simulink model "Cluster_HMI"  (R2024a)
settings: Solver=VariableStepAuto  StartTime=0.0  StopTime=10.0  RelTol=1e-3
libraries: simulink x1, spsMonostableLib x1
settings Model: Creator=henri  LastModifiedBy=henri

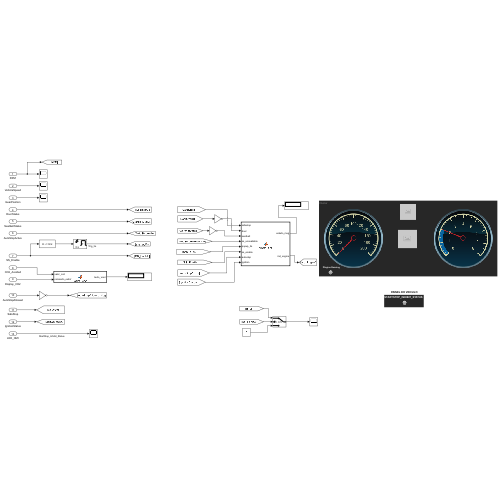
[thumbnail: Simulink's stored preview of the top-level diagram]
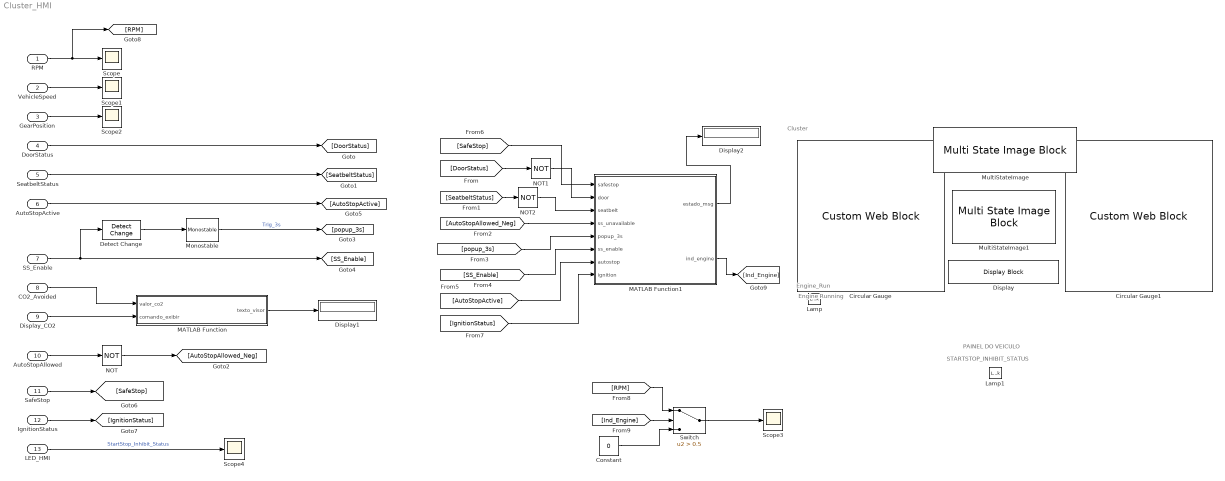
== system Cluster_HMI ==
  note: Engine Running
  note: STARTSTOP_INHIBIT_STATUS
  note: Engine_Run
  note: Cluster
  note: PAINEL DO VEICULO
  RPM : Inport  RequirementInfo={} %GIDa_701cb9d7_1c6a_4930_8ae1_c3f9a837b0c9
  VehicleSpeed : Inport  RequirementInfo={} %GIDa_2d9c3a77_c6f6_418b_8e13_68813d5ea9b5  Port=2
  GearPosition : Inport  RequirementInfo={} %GIDa_c6ce69f4_9c31_429f_b9bc_75ef1a17d6ed  Port=3
  DoorStatus : Inport  RequirementInfo={} %GIDa_d72df632_89b1_4396_adeb_ebc89bf69c51  Port=4
  SeatbeltStatus : Inport  RequirementInfo={} %GIDa_18d845fd_3170_430e_97dc_0ac91aff9f15  Port=5
  AutoStopActive : Inport  RequirementInfo={} %GIDa_37518f2b_e752_4b1f_8c46_cfe48663f65d  Port=6
  SS_Enable : Inport  RequirementInfo={} %GIDa_10efa209_da12_4e26_ab38_1e39670f885c  Port=7
  CO2_Avoided : Inport  RequirementInfo={} %GIDa_176e85e5_0be0_4fa3_869e_c19e09e86116  Port=8
  Display_CO2 : Inport  RequirementInfo={} %GIDa_b6f97d48_dcb8_4ba0_b3dc_e52b49ed6545  Port=9
  AutoStopAllowed : Inport  RequirementInfo={} %GIDa_274fdb3f_b9e4_413b_891d_ddf4024beb1a  Port=10
  SafeStop : Inport  RequirementInfo={} %GIDa_2abc3005_5b3a_47dc_bfb2_0f18a82977d9  Port=11
  IgnitionStatus : Inport  RequirementInfo={} %GIDa_800ccd42_76b0_45b4_b5ac_9e6254392555  Port=12
  LED_HMI : Inport  RequirementInfo={} %GIDa_c1088d5e_6a51_4c66_ba2d_65ca3d813fbb  Port=13
  Circular Gauge : CustomWebBlock  RequirementInfo={} %GIDa_7b8fb6d0_a955_42f4_bee6_c529bf727d9c  LabelPosition=Hide  ShowInitialText=on  Configuration="{\"components\":[{\"name\":\"CircularScaleComponent\",\"settings\":{\"bounds\":{\"max\":200,\"min\":0,\"tickInterval\":20},\"direction\":\"cw\",\"flipLimits\":0,\"innerRadius\":0.75,\"internalTickHeightScaleFactor\":1,\"labelColor\":[255,255,200],\"labelFont\":{\"font\":\"Arial\",\"fontSize\":12},\"labelRadius\":0.528,\"labelTransparency\":1,\"minorTickHeightScaleFactor\":0.2,\"needleImage\":{\"size\":[200,50],\"src\":\"data:image\\/svg+xml;base64,PD94bWwgdmVyc2lvbj0iMS4wIiBlbmNvZGluZz0idXRmLTgiPz4KPCEtLSBHZW5lcmF0b3I6IEFkb2JlIElsbHVzdHJhdG9yIDI0LjEuMiwgU1ZHIEV4cG9ydCBQbHVnLUluIC4gU1ZHIFZlcnNpb246IDYuMDAgQnVpbGQgMCkgIC0tPgo8c3ZnIHZlcnNpb249IjEuMSIgaWQ9IkxheWVyXzEiIHhtbG5zPSJodHRwOi8vd3d3LnczLm9yZy8yMDAwL3N2ZyIgeG1sbnM6eGxpbms9Imh0dHA6Ly93d3cudzMub3JnLzE5OTkveGxpbmsiIHg9IjBweCIgeT0iMHB4IgoJIHZpZXdCb3g9IjAgMCAyMDAgNTAiIHN0eWxlPSJlbmFibGUtYmFja2dyb3VuZDpuZXcgMCAwIDIwMCA1MDsiIHhtbDpzcGFjZT0icHJlc2VydmUiPgo8c3R5bGUgdHlwZT0idGV4dC9jc3MiPgoJLnN0MHtmaWxsOiNFQzIxMjc7fQo8L3N0eWxlPgo8cGF0aCBjbGFzcz0ic3QwIiBkPSJNMTYyLjgsMTMuN0MxNjksNC40LDE4MS43LDEuOSwxOTEsOC4xczExLjgsMTguOSw1LjYsMjguMnMtMTguOSwxMS44LTI4LjIsNS42bDAsMAoJQzE1OS4xLDM1LjYsMTU2LjYsMjMsMTYyLjgsMTMuN0wxNjIuOCwxMy43eiBNMTY1LjgsMTUuOGMtNS4xLDcuNi0zLjEsMTcuOSw0LjYsMjNjNy42LDUuMSwxNy45LDMuMSwyMy00LjYKCWM1LjEtNy42LDMuMS0xNy45LTQuNi0yM2wwLDBDMTgxLjIsNi4yLDE3MC45LDguMiwxNjUuOCwxNS44eiIvPgo8cGF0aCBjbGFzcz0ic3QwIiBkPSJNMC40LDI1Ljl2LTMuM2wxNTktMi41Yy0wLjcsMi42LTAuNyw1LjIsMCw3LjhMMC40LDI1Ljl6Ii8+CjxjaXJjbGUgY2xhc3M9InN0MCIgY3g9IjE3OS42IiBjeT0iMjQiIHI9IjAuNyIvPgo8L3N2Zz4K\"},\"needleOffset\":[0.18464878250906522,0],\"needleOrientation\":-45,\"needleRotation\":180,\"needleSize\":{\"height\":0.11741692305346914,\"width\":0.46108337545091255},\"outerRadius\":0.9,\"position\":[0.05,0.05,0.9,0.9],\"referencePoint\":\"auto\",\"scaleAngle\":270,\"scaleAngleOffset\":135,\"scaleColors\":[],\"scaleColorsSize\":0.2,\"scaleDirection\":\"CW\",\"scalePosition\":[0,0,1,1],\"showLabels\":1,\"showMinorTicks\":1,\"showSpanLine\":1,\"showTicks\":1,\"tickColor\":[252,252,197],\"tickTransparency\":1,\"valueBarColor\":[0,114,189],\"valueBarPosition\":[0,0,1,1],\"valueBarSize\":0.2,\"valueBarTransparency\":1}},{\"name\":\"BackgroundImageComponent\",\"settings\":{\"image\":{\"size\":[500,500],\"src\":\"data:image\\/svg+xml;base64,PD94bWwgdmVyc2lvbj0iMS4wIiBlbmNvZGluZz0iVVRGLTgiIHN0YW5kYWxvbmU9Im5vIj8+CjxzdmcKICAgeG1sbnM6ZGM9Imh0dHA6Ly9wdXJsLm9yZy9kYy9lbGVtZW50cy8xLjEvIgogICB4bWxuczpjYz0iaHR0cDovL2NyZWF0aXZlY29tbW9ucy5vcmcvbnMjIgogICB4bWxuczpyZGY9Imh0dHA6Ly93d3cudzMub3JnLzE5OTkvMDIvMjItcmRmLXN5bnRheC1ucyMiCiAgIHhtbG5zOnN2Zz0iaHR0cDovL3d3dy53My5vcmcvMjAwMC9zdmciCiAgIHhtbG5zPSJodHRwOi8vd3d3LnczLm9yZy8yMDAwL3N2ZyIKICAgeG1sbnM6 ...(+9964 chars)\"},\"position\":[0,0,1,1],\"scaleMode\":\"0\"}},{\"name\":\"ForegroundImageComponent\",\"settings\":{\"image\":{\"size\":[0,0],\"src\":\"default\",\"srcOrientation\":[]},\"isForeground\":1,\"position\":[0,0,1,1],\"scaleMode\":\"0\"}}],\"settings\":{\"BindingType\":\"signal\",\"aspectRatio\":1.032258064516129,\"backgroundColor\":[0,0,0,\"1\"],\"backgroundOffset\":1,\"backgroundOpacity\":1,\"direction\":\"cw\",\"fixedAspectRatio\":\"on\",\"flipLimits\":0,\"orientation\":\"horizontal\",\"showBackgroundColor\":false,\"value\":0,\"version\":\"R2023a\"},\"type\":\"CircularGauge\"}"
  Circular Gauge1 : CustomWebBlock  RequirementInfo={} %GIDa_e85ea3ac_6d53_4628_b3b0_ac8b9261904e  LabelPosition=Hide  ShowInitialText=on  Configuration="{\"components\":[{\"name\":\"CircularScaleComponent\",\"settings\":{\"bounds\":{\"max\":8,\"min\":0,\"tickInterval\":1},\"direction\":\"cw\",\"flipLimits\":0,\"innerRadius\":0.75,\"internalTickHeightScaleFactor\":1,\"labelColor\":[255,255,200],\"labelFont\":{\"font\":\"Arial\",\"fontSize\":12},\"labelRadius\":0.528,\"labelTransparency\":1,\"minorTickHeightScaleFactor\":0.2,\"needleImage\":{\"size\":[200,50],\"src\":\"data:image\\/svg+xml;base64,PD94bWwgdmVyc2lvbj0iMS4wIiBlbmNvZGluZz0idXRmLTgiPz4KPCEtLSBHZW5lcmF0b3I6IEFkb2JlIElsbHVzdHJhdG9yIDI0LjEuMiwgU1ZHIEV4cG9ydCBQbHVnLUluIC4gU1ZHIFZlcnNpb246IDYuMDAgQnVpbGQgMCkgIC0tPgo8c3ZnIHZlcnNpb249IjEuMSIgaWQ9IkxheWVyXzEiIHhtbG5zPSJodHRwOi8vd3d3LnczLm9yZy8yMDAwL3N2ZyIgeG1sbnM6eGxpbms9Imh0dHA6Ly93d3cudzMub3JnLzE5OTkveGxpbmsiIHg9IjBweCIgeT0iMHB4IgoJIHZpZXdCb3g9IjAgMCAyMDAgNTAiIHN0eWxlPSJlbmFibGUtYmFja2dyb3VuZDpuZXcgMCAwIDIwMCA1MDsiIHhtbDpzcGFjZT0icHJlc2VydmUiPgo8c3R5bGUgdHlwZT0idGV4dC9jc3MiPgoJLnN0MHtmaWxsOiNFQzIxMjc7fQo8L3N0eWxlPgo8cGF0aCBjbGFzcz0ic3QwIiBkPSJNMTYyLjgsMTMuN0MxNjksNC40LDE4MS43LDEuOSwxOTEsOC4xczExLjgsMTguOSw1LjYsMjguMnMtMTguOSwxMS44LTI4LjIsNS42bDAsMAoJQzE1OS4xLDM1LjYsMTU2LjYsMjMsMTYyLjgsMTMuN0wxNjIuOCwxMy43eiBNMTY1LjgsMTUuOGMtNS4xLDcuNi0zLjEsMTcuOSw0LjYsMjNjNy42LDUuMSwxNy45LDMuMSwyMy00LjYKCWM1LjEtNy42LDMuMS0xNy45LTQuNi0yM2wwLDBDMTgxLjIsNi4yLDE3MC45LDguMiwxNjUuOCwxNS44eiIvPgo8cGF0aCBjbGFzcz0ic3QwIiBkPSJNMC40LDI1Ljl2LTMuM2wxNTktMi41Yy0wLjcsMi42LTAuNyw1LjIsMCw3LjhMMC40LDI1Ljl6Ii8+CjxjaXJjbGUgY2xhc3M9InN0MCIgY3g9IjE3OS42IiBjeT0iMjQiIHI9IjAuNyIvPgo8L3N2Zz4K\"},\"needleOffset\":[0.18464878250906522,0],\"needleOrientation\":-45,\"needleRotation\":180,\"needleSize\":{\"height\":0.11741692305346914,\"width\":0.46108337545091255},\"outerRadius\":0.9,\"position\":[0.05,0.05,0.9,0.9],\"referencePoint\":\"auto\",\"scaleAngle\":270,\"scaleAngleOffset\":135,\"scaleColors\":[],\"scaleColorsSize\":0.2,\"scaleDirection\":\"CW\",\"scalePosition\":[0,0,1,1],\"showLabels\":1,\"showMinorTicks\":1,\"showSpanLine\":1,\"showTicks\":1,\"tickColor\":[252,252,197],\"tickTransparency\":1,\"valueBarColor\":[0,114,189],\"valueBarPosition\":[0,0,1,1],\"valueBarSize\":0.2,\"valueBarTransparency\":1}},{\"name\":\"BackgroundImageComponent\",\"settings\":{\"image\":{\"size\":[500,500],\"src\":\"data:image\\/svg+xml;base64,PD94bWwgdmVyc2lvbj0iMS4wIiBlbmNvZGluZz0iVVRGLTgiIHN0YW5kYWxvbmU9Im5vIj8+CjxzdmcKICAgeG1sbnM6ZGM9Imh0dHA6Ly9wdXJsLm9yZy9kYy9lbGVtZW50cy8xLjEvIgogICB4bWxuczpjYz0iaHR0cDovL2NyZWF0aXZlY29tbW9ucy5vcmcvbnMjIgogICB4bWxuczpyZGY9Imh0dHA6Ly93d3cudzMub3JnLzE5OTkvMDIvMjItcmRmLXN5bnRheC1ucyMiCiAgIHhtbG5zOnN2Zz0iaHR0cDovL3d3dy53My5vcmcvMjAwMC9zdmciCiAgIHhtbG5zPSJodHRwOi8vd3d3LnczLm9yZy8yMDAwL3N2ZyIKICAgeG1sbnM6 ...(+9964 chars)\"},\"position\":[0,0,1,1],\"scaleMode\":\"0\"}},{\"name\":\"ForegroundImageComponent\",\"settings\":{\"image\":{\"size\":[0,0],\"src\":\"default\",\"srcOrientation\":[]},\"isForeground\":1,\"position\":[0,0,1,1],\"scaleMode\":\"0\"}}],\"settings\":{\"BindingType\":\"signal\",\"aspectRatio\":1.032258064516129,\"backgroundColor\":[0,0,0,\"1\"],\"backgroundOffset\":1,\"backgroundOpacity\":1,\"direction\":\"cw\",\"fixedAspectRatio\":\"on\",\"flipLimits\":0,\"orientation\":\"horizontal\",\"showBackgroundColor\":false,\"value\":0,\"version\":\"R2023a\"},\"type\":\"CircularGauge\"}"
  Constant : Constant  RequirementInfo={} %GIDa_7eaddd39_03fd_4774_8ce7_06ac99342a11  Value=0
  Detect Change : simulink/Logic and Bit Operations/Detect Change  vinit=0  OutDataTypeStr=boolean
  Display : DisplayBlock  RequirementInfo={} %GIDa_aa89c4e3_5f39_4481_9063_9e987de78835  LabelPosition=Hide  Transparency=1
  Display1 : Display
      settings: RequirementInfo={} %GIDa_3383fe43_73fa_45f6_bd7d_58d124f59e38
  Display2 : Display
      settings: RequirementInfo={} %GIDa_40a4ffce_79c5_466a_a116_50932f87ad3b
  Lamp : LampBlock  RequirementInfo={} %GIDa_584dc557_8e58_4761_ad30_6086ceb2bee4  LabelPosition=Hide
  Lamp1 : LampBlock  RequirementInfo={} %GIDa_19e065cc_f85f_4edf_b463_5f27953babfd  LabelPosition=Hide
  MATLAB Function : MATLAB Function  RequirementInfo={} %GIDa_0a7b60b7_ce26_4871_a736_41ae8e450be9  TreatAsAtomicUnit=on
  MATLAB Function1 : MATLAB Function  RequirementInfo={} %GIDa_19d8ed7e_de69_4d18_8458_21e93ce7cd2d  TreatAsAtomicUnit=on
  Monostable : spsMonostableLib/Monostable  EdgeDetect=Rising  PulseDuration=3  ic=0  Ts=0
      settings: LibrarySourceBlock=sps_lib/Control/Monostable
  MultiStateImage : MultiStateImageBlock  RequirementInfo={} %GIDa_662be9bc_8bef_443d_9e81_c1b2cdb77985  LabelPosition=Hide
  MultiStateImage1 : MultiStateImageBlock  RequirementInfo={} %GIDa_5e01354f_4671_4b86_9fde_4ed7b7aa1971  LabelPosition=Hide
  NOT : Logic  RequirementInfo={} %GIDa_81d60eac_65d1_4224_906b_b6edff622eda  Operator=NOT  IconShape=distinctive  AllPortsSameDT=off  OutDataTypeStr=boolean
  NOT1 : Logic  RequirementInfo={} %GIDa_da543115_b6c1_4c08_8c22_51fdf42d67fd  Operator=NOT  IconShape=distinctive  AllPortsSameDT=off  OutDataTypeStr=boolean
  NOT2 : Logic  RequirementInfo={} %GIDa_2b656ab1_76fb_4310_941e_5bc774d4b54f  Operator=NOT  IconShape=distinctive  AllPortsSameDT=off  OutDataTypeStr=boolean
  Scope{,1..4} (5 alike) : Scope
      Scope settings: RequirementInfo={} %GIDa_bd9bb622_bd6e_4b97_9f6e_72145f6f1df7
      Scope1 settings: RequirementInfo={} %GIDa_8237f8ec_35d9_404e_9e4c_66062df8a6b6
      Scope2 settings: RequirementInfo={} %GIDa_79327c20_79b8_42b8_9cad_ed2392b7937b
      Scope3 settings: RequirementInfo={} %GIDa_7a1ee26b_76fb_497e_a582_85f790c6cb47
      Scope4 settings: RequirementInfo={} %GIDa_ae7f9845_f57c_408a_bcfe_ca6ab02a3b36
  Switch : Switch  RequirementInfo={} %GIDa_510e6e19_78a9_425c_8587_97d427917c88  Criteria=u2 > Threshold  Threshold=0.5  SaturateOnIntegerOverflow=off  InputSameDT=off
  wires:
  [Ind_Engine] -> Switch/2
  Detect Change/1 -> Monostable/1
  MATLAB Function1/2(ind_engine) -> [Ind_Engine]
  Switch/1 -> Scope3/1
  [AutoStopActive] -> MATLAB Function1/7(autostop)
  Constant/1 -> Switch/3
  [SeatbeltStatus] -> NOT2/1
  Display_CO2/1 -> MATLAB Function/2(comando_exibir)
  Monostable/1 -> [popup_3s]  "Trig_3s"
  NOT2/1 -> MATLAB Function1/3(seatbelt)
  MATLAB Function1/1(estado_msg) -> Display2/1
  [IgnitionStatus] -> MATLAB Function1/8(ignition)
  VehicleSpeed/1 -> Scope1/1
  SafeStop/1 -> [SafeStop]
  [AutoStopAllowed_Neg] -> MATLAB Function1/4(ss_unavailable)
  NOT1/1 -> MATLAB Function1/2(door)
  [DoorStatus] -> NOT1/1
  MATLAB Function/1(texto_visor) -> Display1/1
  [SafeStop] -> MATLAB Function1/1(safestop)
  LED_HMI/1 -> Scope4/1  "StartStop_Inhibit_Status"
  RPM/1 -> [RPM], Scope/1
  IgnitionStatus/1 -> [IgnitionStatus]
  SS_Enable/1 -> Detect Change/1, [SS_Enable]
  [RPM] -> Switch/1
  DoorStatus/1 -> [DoorStatus]
  [SS_Enable] -> MATLAB Function1/6(ss_enable)
  AutoStopAllowed/1 -> NOT/1
  CO2_Avoided/1 -> MATLAB Function/1(valor_co2)
  [popup_3s] -> MATLAB Function1/5(popup_3s)
  AutoStopActive/1 -> [AutoStopActive]
  NOT/1 -> [AutoStopAllowed_Neg]
  SeatbeltStatus/1 -> [SeatbeltStatus]
  GearPosition/1 -> Scope2/1

== matlab function Cluster_HMI/MATLAB Function1 ==
  data: safestop input; door input; estado_msg output; seatbelt input; ss_unavailable input; popup_3s input; ss_enable input; autostop input; ignition input; ind_engine output
function [estado_msg, ind_engine] = arbitro_hmi(safestop, door, seatbelt, ss_unavailable, popup_3s, ss_enable, autostop, ignition)
    
    % --- LÓGICA DO LAMP (Motor Running vs Off) ---
    % O motor só está rodando (1) se a ignição estiver ligada, 
    % e o sistema não tiver desligado o motor (autostop ou safestop).
    if (ignition == 1) && (autostop == 0) && (safestop == 0)
        ind_engine = 1; % Motor Ligado (Lamp ON)
    else
        ind_engine = 0; % Motor Desligado (Lamp OFF)
    end

    % --- LÓGICA DO CLUSTER CENTRAL (Mensagens) ---
    estado_msg = 0; % Tela Limpa
    
    % PRIORIDADE ZERO: Bloqueio de Segurança (Safe Stop)
    if safestop == 1
        estado_msg = 7; 
        
    % PRIORIDADE 1: Falhas e Segurança (Crítico)
    elseif door == 1
        estado_msg = 1; 
        
    elseif seatbelt == 1 
        estado_msg = 2; 
        
    % PRIORIDADE 2: Pop-up Temporário
    elseif popup_3s == 1
        if ss_enable == 1
            estado_msg = 4; 
        else
            estado_msg = 5; 
        end
        
    % PRIORIDADE 3: Operação Normal (AutoStop)
    elseif autostop == 1
        estado_msg = 6; 
        
    % PRIORIDADE 4: Sistema Indisponível (Laranja)
    elseif ss_unavailable == 1 && autostop == 0 && ss_enable == 1
        estado_msg = 3; 
    end
end

== matlab function Cluster_HMI/MATLAB Function ==
  data: valor_co2 input; texto_visor output; comando_exibir input
function texto_visor = logica_co2(valor_co2, comando_exibir)
    % O Simulink exige que o número seja inteiro (round) para virar string
    if comando_exibir == 1
        texto_visor = string(round(valor_co2)) + " g CO2 Evitado";
    else
        texto_visor = ""; 
    end
end
